simulink model "Q8_Simulink"  (R2019b)
settings: Solver=VariableStepAuto  StartTime=0.0  StopTime=10.0  RelTol=1e-3
undefined symbols (not defined in the file): C, Cref, d, E_x, E_y, F, G, Kc, theta_3_ref, Ts
settings Model: Creator=mfust  LastModifiedBy=mfust

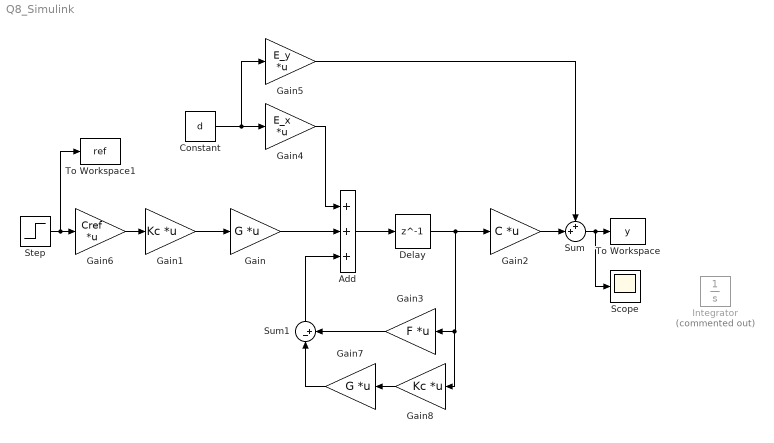
== system Q8_Simulink ==
  Add : Sum  Inputs=+++
  Constant : Constant  Value=d
  Delay : Delay  DelayLength=1  InitialCondition=[0 0 0 0 0 0]'  SampleTime=Ts
  Gain : Gain  Gain=G  Multiplication=Matrix(K*u)
  Gain1 : Gain  Gain=Kc  Multiplication=Matrix(K*u)
  Gain2 : Gain  Gain=C  Multiplication=Matrix(K*u)
  Gain3 : Gain  Gain=F  Multiplication=Matrix(K*u)
  Gain4 : Gain  Gain=E_x  Multiplication=Matrix(K*u)
  Gain5 : Gain  Gain=E_y  Multiplication=Matrix(K*u)
  Gain6 : Gain  Gain=Cref  Multiplication=Matrix(K*u)
  Gain7 : Gain  Gain=G  Multiplication=Matrix(K*u)
  Gain8 : Gain  Gain=Kc  Multiplication=Matrix(K*u)
  Integrator : Integrator  Commented=on  InitialCondition=[0 0 0 0 0 0]'
  Scope : Scope
  Step : Step  After=theta_3_ref  SampleTime=0
  Sum : Sum  Inputs=++|
  Sum1 : Sum  Inputs=|-+
  To Workspace : ToWorkspace  VariableName=y  SaveFormat=Structure With Time  SampleTime=-1
  To Workspace1 : ToWorkspace  VariableName=ref  SaveFormat=Structure With Time  SampleTime=-1
  wires:
  Add/1 -> Delay/1
  Delay/1 -> Gain8/1, Gain3/1, Gain2/1
  Gain4/1 -> Add/1
  Constant/1 -> Gain5/1, Gain4/1
  Gain2/1 -> Sum/2
  Gain5/1 -> Sum/1
  Sum/1 -> Scope/1, To Workspace/1
  Gain6/1 -> Gain1/1
  Gain/1 -> Add/2
  Step/1 -> To Workspace1/1, Gain6/1
  Gain3/1 -> Sum1/2
  Sum1/1 -> Add/3
  Gain1/1 -> Gain/1
  Gain7/1 -> Sum1/1
  Gain8/1 -> Gain7/1
